simulink model "FanTuner"  (R2019a)
settings: Solver=VariableStepAuto  StartTime=0.0  StopTime=100  RelTol=1e-3
undefined symbols (not defined in the file or in its folder): k
libraries: simulink x1
settings Model: Creator=hermanko  LastModifiedBy=hermanko

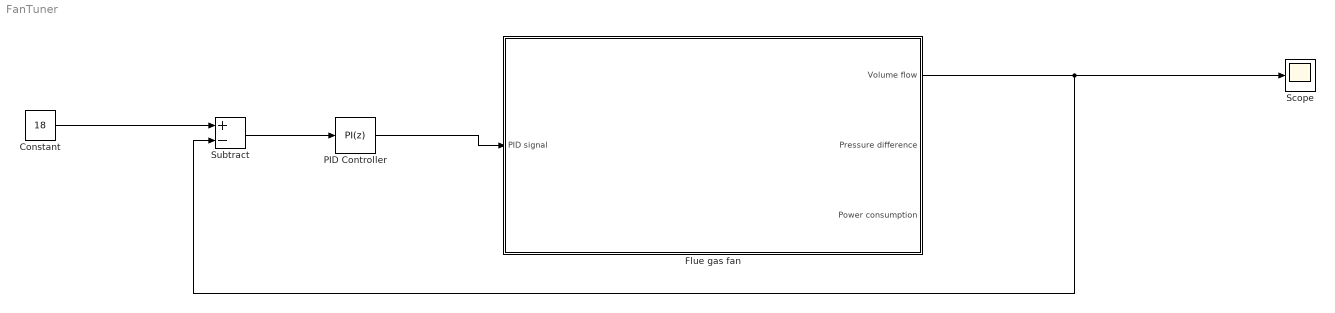
== system FanTuner ==
  Constant : Constant  Value=18
  Flue gas fan : Subsystem
  PID Controller : simulink/Continuous/PID Controller  Controller=PI  Form=Parallel  TimeDomain=Discrete-time  SampleTime=1  IntegratorMethod=Forward Euler  FilterMethod=Forward Euler  ControllerParametersSource=internal  P=15  I=15  D=0  UseFilter=on  N=100  TunerSelectOption=Transfer Function Based (PID Tuner App)  InitialConditionSource=internal  InitialConditionForIntegrator=1.66e+03  InitialConditionForFilter=0  DifferentiatorICPrevScaledInput=0  ExternalReset=none  TrackingMode=off  Kt=1  LimitOutput=off  UpperSaturationLimit=inf  LowerSaturationLimit=-inf  LinearizeAsGain=on  AntiWindupMode=none  Kb=1  POutMin=[]  POutMax=[]  IOutMin=[]  IOutMax=[]  DOutMin=[]  DOutMax=[]  NOutMin=[]  NOutMax=[]  SumOutMin=[]  SumOutMax=[]  SaturationOutMin=[]  SaturationOutMax=[]  PParamMin=[]  PParamMax=[]  IParamMin=[]  IParamMax=[]  DParamMin=[]  DParamMax=[]  NParamMin=[]  NParamMax=[]  KbParamMin=[]  KbParamMax=[]  KtParamMin=[]  KtParamMax=[]  KbOutMin=[]  KbOutMax=[]  KtOutMin=[]  KtOutMax=[]  IntegratorOutMin=[]  IntegratorOutMax=[]  FilterOutMin=[]  FilterOutMax=[]  SumI1OutMin=[]  SumI1OutMax=[]  SumI2OutMin=[]  SumI2OutMax=[]  SumI3OutMin=[]  SumI3OutMax=[]  SumI4OutMin=[]  SumI4OutMax=[]  SumDOutMin=[]  SumDOutMax=[]  DifferentiatorOutMin=[]  DifferentiatorOutMax=[]  FilterDiffOutCoefMin=[]  FilterDiffOutCoefMax=[]  ReciprocalOutMin=[]  ReciprocalOutMax=[]  SumDenOutMin=[]  SumDenOutMax=[]  SumNumOutMin=[]  SumNumOutMax=[]  DivideOutMin=[]  DivideOutMax=[]  IntegratorContinuousStateAttributes=''  IntegratorStateMustResolveToSignalObject=off  IntegratorRTWStateStorageClass=Auto  FilterContinuousStateAttributes=''  FilterStateMustResolveToSignalObject=off  FilterRTWStateStorageClass=Auto  ParallelPVariant=InternalParameters  IdealPVariant=Disabled  IVariant=InternalParameters  DVariant=Disabled  IntegratorVariant=Discrete  SatVariant=Disabled  AWVariant=Passthrough  PCopyVariant=Disabled  TRVariant=Disabled  FdbkBlocksVariant=Forward  IdealPFdbkVariant=Disabled  SatFdbkVariant=Disabled  DerivativeFilterVariant=Disabled  NVariant=Disabled  NCopyVariant=Disabled_SignalSpec  FilterICVariant=Disabled  IntegratorICVariant=InternalICs  ExternalResetVariant=Disabled  TRSumVariant=Passthrough  SumFdbkVariant=Disabled  SumVariant=Sum_PI
  Scope : Scope
  Subtract : Sum  Inputs=+-
  wires:
  PID Controller/1 -> Flue gas fan/1(PID signal)
  Flue gas fan/1(Volume flow) -> Subtract/2, Scope/1
  Constant/1 -> Subtract/1
  Subtract/1 -> PID Controller/1

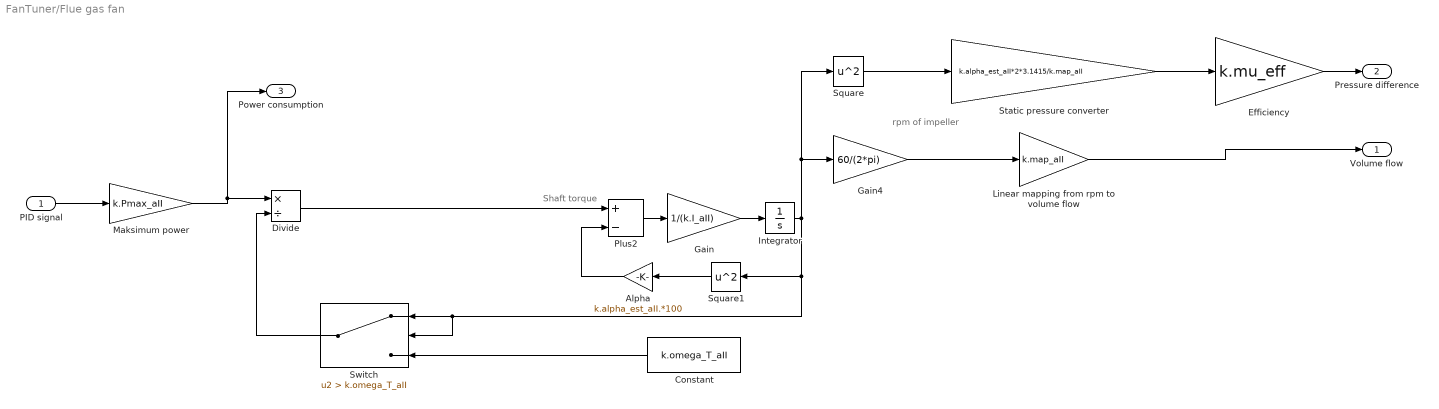
== system FanTuner/Flue gas fan ==
  note: rpm of impeller
  note: Shaft torque
  PID signal : Inport
  Alpha : Gain  Gain=k.alpha_est_aII.*100
  Constant : Constant  Value=k.omega_T_aII
  Divide : Product  Inputs=*/
  Efficiency : Gain  Gain=k.mu_eff
  Gain : Gain  Gain=1/(k.I_aII)
  Gain4 : Gain  Gain=60/(2*pi)
  Integrator : Integrator
  "Linear mapping from rpm to volume flow " : Gain  Gain=k.map_aII
  "Maksimum power " : Gain  Gain=k.Pmax_aII
  Plus2 : Sum  Inputs=+-
  Square : Math  Operator=square  SaturateOnIntegerOverflow=on
  Square1 : Math  Operator=square  SaturateOnIntegerOverflow=on
  Static pressure converter : Gain  Gain=k.alpha_est_aII*2*3.1415/k.map_aII
  Switch : Switch  Criteria=u2 > Threshold  Threshold=k.omega_T_aII
  Volume flow : Outport
  Pressure difference : Outport  Port=2
  Power consumption : Outport  Port=3
  wires:
  Integrator/1 -> Square/1, Gain4/1, Switch/2, Switch/1, Square1/1
  Divide/1 -> Plus2/1
  Gain4/1 -> "Linear mapping from rpm to volume flow "/1
  Square/1 -> Static pressure converter/1
  Efficiency/1 -> Pressure difference/1
  "Maksimum power "/1 -> Power consumption/1, Divide/1
  Static pressure converter/1 -> Efficiency/1
  Alpha/1 -> Plus2/2
  Square1/1 -> Alpha/1
  Gain/1 -> Integrator/1
  Plus2/1 -> Gain/1
  PID signal/1 -> "Maksimum power "/1
  "Linear mapping from rpm to volume flow "/1 -> Volume flow/1
  Switch/1 -> Divide/2
  Constant/1 -> Switch/3
